simulink subsystem "one_axis_sun_sensor_model"  (R2024a)
settings: Solver=VariableStepAuto  StartTime=0.0  StopTime=10.0  RelTol=1e-3
settings Model: Creator=joshu  LastModifiedBy=joshu

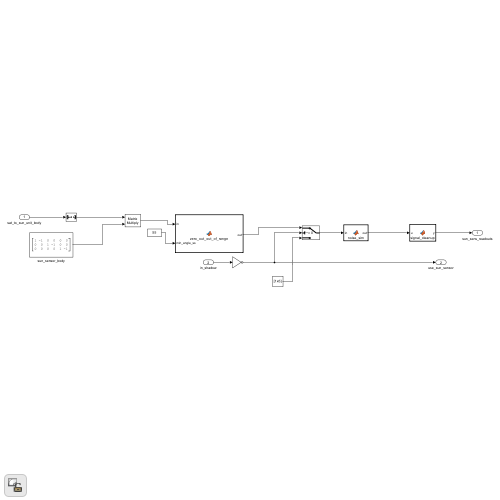
[thumbnail: Simulink's stored preview of the top-level diagram]
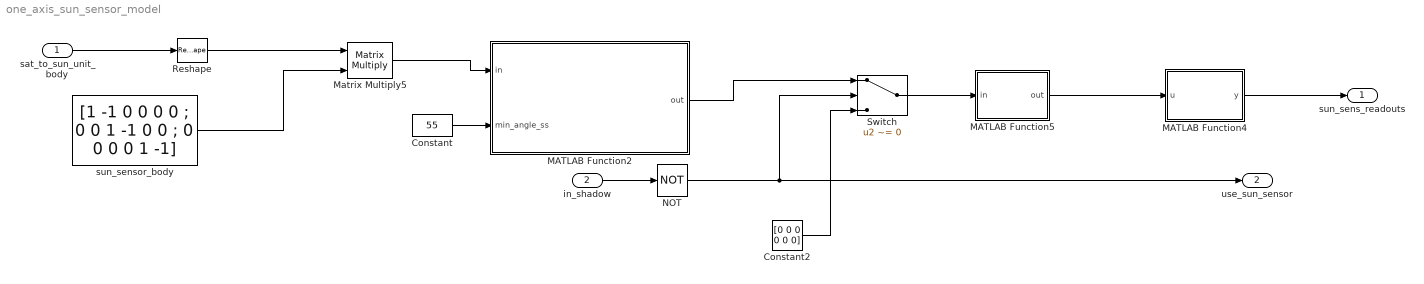
== system one_axis_sun_sensor_model ==
  sat_to_sun_unit_body : Inport
  in_shadow : Inport  Port=2
  Constant : Constant  Value=55
  Constant2 : Constant  Value=[0 0 0 0 0 0]  VectorParams1D=off
  MATLAB Function2 : MATLAB Function  TreatAsAtomicUnit=on
  MATLAB Function4 : MATLAB Function  TreatAsAtomicUnit=on
  MATLAB Function5 : MATLAB Function  TreatAsAtomicUnit=on
  Matrix Multiply5 : Product  Multiplication=Matrix(*)
  NOT : Logic  Operator=NOT  IconShape=distinctive  AllPortsSameDT=off  OutDataTypeStr=boolean
  Reshape : Reshape  OutputDimensionality=Row vector (2-D)
  Switch : Switch  Criteria=u2 ~= 0  SaturateOnIntegerOverflow=off  InputSameDT=off
  sun_sensor_body : Constant  Value=[1 -1 0 0 0 0 ; 0 0 1 -1 0 0 ; 0 0 0 0 1 -1]
  sun_sens_readouts : Outport
  use_sun_sensor : Outport  Port=2
  wires:
  Matrix Multiply5/1 -> MATLAB Function2/1(in)
  MATLAB Function5/1(out) -> MATLAB Function4/1(u)
  Constant/1 -> MATLAB Function2/2(min_angle_ss)
  Reshape/1 -> Matrix Multiply5/1
  MATLAB Function4/1(y) -> sun_sens_readouts/1
  MATLAB Function2/1(out) -> Switch/1
  sat_to_sun_unit_body/1 -> Reshape/1
  sun_sensor_body/1 -> Matrix Multiply5/2
  Switch/1 -> MATLAB Function5/1(in)
  Constant2/1 -> Switch/3
  in_shadow/1 -> NOT/1
  NOT/1 -> Switch/2, use_sun_sensor/1

== matlab function one_axis_sun_sensor_model/MATLAB Function4 ==
  data: u input; y output
function y = signal_cleanup(u)
y = [0,0,0];

if u(1) == 0
    y(1) = -u(2);
else
    y(1) = u(1);
end

if u(3) == 0
    y(2) = -u(4);
else
    y(2) = u(3);
end

if u(5) == 0
    y(3) = -u(6);
else
    y(3) = u(5);
end


end

== matlab function one_axis_sun_sensor_model/MATLAB Function5 ==
  settings: updateMethod=DISCRETE
  data: in input; out output
function out = noise_sim(in)

    out = in;

    for i = 1:length(out)
        sgn = sign(out(i));
        ang = acosd(abs(out(i)));
        if ang <= 45
            %out(i) = cosd(ang + (rand()*0.6-0.3))*sgn;
        elseif ang <= 60
            %out(i) = cosd(ang + (rand()*1.2-0.6))*sgn;
        end
    end

== matlab function one_axis_sun_sensor_model/MATLAB Function2 ==
  data: in input; out output; min_angle_ss input
function out = zero_out_out_of_range(in, min_angle_ss)
    
    min_value = cosd(min_angle_ss);
    out = in;
    for i = 1:length(out)
        if out(i) < min_value
            out(i) = 0;
        end
    end
